simulink model "band_begr_rausch1"  (Simulink 7.8)
settings: Solver=ode45  StartTime=0.0  StopTime=10.0  RelTol=1e-3
undefined symbols (not defined in the file or in its folder): Fs, get, sided, Two
libraries: simulink x1, dspstat3 x1, dspsnks4 x1
settings Model: Creator=josef  LastModifiedBy=josef

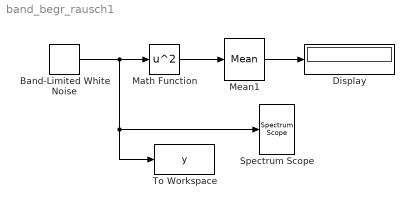
== system band_begr_rausch1 ==
  Band-Limited White Noise : simulink/Sources/Band-Limited White Noise  Cov=[1/10000]  Ts=1/10000  seed=[23341]
  Display : Display
  Math Function : Math  Operator=square  SaturateOnIntegerOverflow=on
  Mean1 : dspstat3/Mean  run=on  reset_popup=None  InputProcessing=Inherited (this choice will be removed - see release notes)  directionMode=Each column  dimension=1  treatSBRowAsCol=on  roiEnable=off  roiType=Rectangles  roiPortion=Entire ROI  roiOutput=Individual statistics for each ROI  roiFlag=off  outputDataTypeStr=Inherit: Same as accumulator  outputLastDataTypeStr=Inherit: Same as accumulator  outputMin=[]  outputMax=[]  roundingMode=Floor  overflowMode=off
  Spectrum Scope : dspsnks4/Spectrum Scope  ScopeProperties=on  Domain=Frequency  HorizSpan=1  UseBuffer=on  BufferSize=256  Overlap=0  TreatMby1Signals=One channel  inpFftLenInherit=on  FFTlength=256  numAvg=100  DisplayProperties=off  AxisGrid=on  Memory=off  FrameNumber=on  AxisLegend=off  AxisZoom=off  OpenScopeAtSimStart=on  OpenScopeImmediately=off  FigPos=get(0,'defaultfigureposition')  AxisProperties=off  XUnits=Hertz  XRange=Two-sided ((-Fs/2...Fs/2])  XDisplay=0  InheritXIncr=on  XIncr=1.0  XLabel=Samples  XLimit=User-defined  YUnits=dBW/Hertz  XMax=5000  XMin=-5000  YLabel=Magnitude-squared, dB  LineProperties=off  wintypeSpecScope=Hamming  RsSpecScope=50  betaSpecScope=5  winsampSpecScope=Symmetric  XAxisParamsVer=6.9  isFrameUpgraded=on
      settings: YMin=-44.4758  YMax=-37.3159
  To Workspace : ToWorkspace  VariableName=y  SampleTime=-1  SaveFormat=Array
  wires:
  Math Function/1 -> Mean1/1
  Mean1/1 -> Display/1
  Band-Limited White Noise/1 -> Math Function/1, Spectrum Scope/1, To Workspace/1
